simulink model "SyncGen_with_Grid_controll"  (R2013a)
settings: Solver=ode23  StartTime=2  StopTime=10  FixedStep=10^-3  MaxStep=1e-2  RelTol=1e-2
undefined symbols (not defined in the file): J, L_g, R_g, R_l
libraries: powerlib x18, powerlib_meascontrol x4, SyncGenLib x1
settings Model: Creator=Elad  LastModifiedBy=USER
settings DataIOCC: SignalLoggingSaveFormat=ModelDataLogs
settings DebuggingCC: MultiTaskDSMMsg=warning  MultiTaskCondExecSysMsg=none  StateNameClashWarn=none  StrictBusMsg=None
settings RTWCC: IncludeERTFirstTime=on

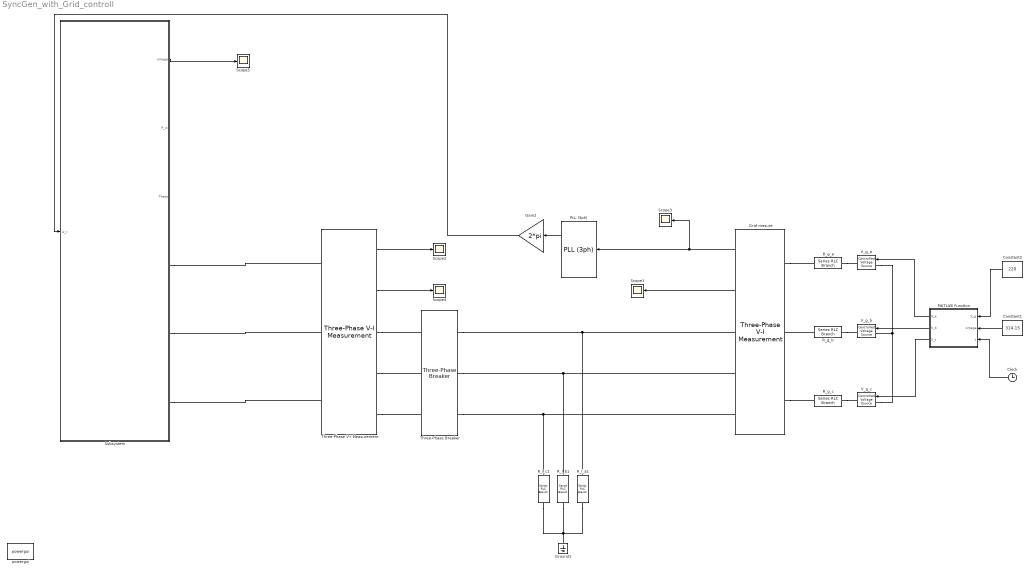
== system SyncGen_with_Grid_controll ==
  Clock : Clock
  Constant1 : Constant  Value=314.15
  Constant2 : Constant  Value=220
  Gain2 : Gain  Gain=2*pi
  Grid mesure : powerlib/Measurements/Three-Phase V-I Measurement  VoltageMeasurement=phase-to-ground  SetLabelV=off  LabelV=Vabc  Vpu=off  VpuLL=off  CurrentMeasurement=yes  SetLabelI=off  LabelI=Iabc  Ipu=off  Pbase=100e6  Vbase=500e3  OutputType=Complex  PhasorSimulation=off  PSBequivalent=0
  Ground1 : powerlib/Elements/Ground  LConnTagsString=a
  MATLAB Function : MATLAB Function  TreatAsAtomicUnit=on
  PLL (3ph) : powerlib_meascontrol/PLL/PLL (3ph)  Fmin=45  Par_Init=[0, 60]  ParK=[180, 3200, 1]  TcD=1e-4  MaxRateChangeFreq=12  FilterCutOffFreq=25  Ts=0  AGC=on
  R_g_a : powerlib/Elements/Series RLC Branch  LConnTagsString=__new0  RConnTagsString=__new0  BranchType=RL  Resistance=R_g  Inductance=L_g  SetiL0=off  InitialCurrent=0  Capacitance=1e-6  Setx0=off  InitialVoltage=0  Measurements=None
  R_g_b : powerlib/Elements/Series RLC Branch  LConnTagsString=__new0  RConnTagsString=__new0  BranchType=RL  Resistance=R_g  Inductance=L_g  SetiL0=off  InitialCurrent=0  Capacitance=1e-6  Setx0=off  InitialVoltage=0  Measurements=None
  R_g_c : powerlib/Elements/Series RLC Branch  LConnTagsString=__new0  RConnTagsString=__new0  BranchType=RL  Resistance=R_g  Inductance=L_g  SetiL0=off  InitialCurrent=0  Capacitance=1e-6  Setx0=off  InitialVoltage=0  Measurements=None
  R_l_a1 : powerlib/Elements/Series RLC Branch  LConnTagsString=__new0  RConnTagsString=__new0  BranchType=R  Resistance=R_l  Inductance=1e-3  SetiL0=off  InitialCurrent=0  Capacitance=1e-6  Setx0=off  InitialVoltage=0  Measurements=None
  R_l_b1 : powerlib/Elements/Series RLC Branch  LConnTagsString=__new0  RConnTagsString=__new0  BranchType=R  Resistance=R_l  Inductance=1e-3  SetiL0=off  InitialCurrent=0  Capacitance=1e-6  Setx0=off  InitialVoltage=0  Measurements=None
  R_l_c1 : powerlib/Elements/Series RLC Branch  LConnTagsString=__new0  RConnTagsString=__new0  BranchType=R  Resistance=R_l  Inductance=1e-3  SetiL0=off  InitialCurrent=0  Capacitance=1e-6  Setx0=off  InitialVoltage=0  Measurements=None
  Scope{1..5} (5 alike) : Scope
      Scope1 settings: TimeRange=5  YMin=-0.11  YMax=0.11
      Scope2 settings: TimeRange=8  YMin=-12.5  YMax=15
      Scope3 settings: TimeRange=5  YMin=-200  YMax=225  SaveName=ScopeData3
      Scope4 settings: TimeRange=5  YMin=-0.005  YMax=0.005  SaveName=ScopeData4
      Scope5 settings: TimeRange=5  YMin=293  YMax=316  SaveName=ScopeData2
  Subsystem : Subsystem
  Three-Phase V-I Measurement : powerlib/Measurements/Three-Phase V-I Measurement  VoltageMeasurement=phase-to-ground  SetLabelV=off  LabelV=Vabc  Vpu=off  VpuLL=off  CurrentMeasurement=yes  SetLabelI=off  LabelI=Iabc  Ipu=off  Pbase=100e6  Vbase=500e3  OutputType=Complex  PhasorSimulation=off  PSBequivalent=0
  Three-Phase Breaker : powerlib/Elements/Three-Phase Breaker  InitialState=open  SwitchA=on  SwitchB=on  SwitchC=on  SwitchTimes=[5]  External=off  BreakerResistance=0.001  SnubberResistance=1e6  SnubberCapacitance=inf  Measurements=None
  V_g_a : powerlib/Electrical Sources/Controlled Voltage Source  Initialize=off  Source_Type=AC  Amplitude=0  Phase=0  Frequency=0  Measurements=None
  V_g_b : powerlib/Electrical Sources/Controlled Voltage Source  Initialize=off  Source_Type=AC  Amplitude=0  Phase=0  Frequency=0  Measurements=None
  V_g_c : powerlib/Electrical Sources/Controlled Voltage Source  Initialize=off  Source_Type=AC  Amplitude=0  Phase=0  Frequency=0  Measurements=None
  powergui : powerlib/powergui  Priority=1  SimulationMode=Continuous  SolverType=Tustin  SampleTime=50e-6  frequency=60  SPID=off  DisableSnubberDevices=off  DisableRonSwitches=off  DisableVfSwitches=off  SwTol=0  Interpol=off  DisplayEquations=off  frequencyindice=0  Pbase=100e6  ErrMax=1e-4  Iterations=50  UnitsV=kV  UnitsW=MW  FunctionMessages=off  echomessages=off  HookPort=off  EnableUseOfTLC=off  x0status=blocks  RestoreLinks=warning  ResistiveCurrentMeasurement=off  Frange=[0:2:500]  Ylog=off  Xlog=on  ShowGrid=off  save=off  variable=ZData  ZoomFFT=off  StartTime=0.0  cycles=1  DisplayStyle=1  fundamental=60  FreqAxis=off  MaxFrequency=1000  frequencyindicesteady=1  RmsSteady=1  display=off  Ts=0  methode=off
  wires:
  Three-Phase V-I Measurement/1 -> Scope2/1
  Three-Phase V-I Measurement/2 -> Scope4/1
  Subsystem/1(omega) -> Scope5/1
  MATLAB Function/1(V_a) -> V_g_a/1
  MATLAB Function/2(V_b) -> V_g_b/1
  MATLAB Function/3(V_c) -> V_g_c/1
  Constant1/1 -> MATLAB Function/2(omega)
  Constant2/1 -> MATLAB Function/1(V_g)
  Clock/1 -> MATLAB Function/3(t)
  Grid mesure/2 -> Scope1/1
  Grid mesure/1 -> Scope3/1, PLL (3ph)/1
  PLL (3ph)/1 -> Gain2/1
  Gain2/1 -> Subsystem/1(w_r)
  connections:
  V_g_a/LConn1 -- V_g_b/LConn1 -- V_g_c/LConn1
  R_l_b1/RConn1 -- R_l_a1/RConn1 -- Ground1/LConn1 -- R_l_c1/RConn1
  Grid mesure/RConn2 -- Three-Phase Breaker/RConn2 -- R_l_b1/LConn1
  Grid mesure/RConn3 -- R_l_c1/LConn1 -- Three-Phase Breaker/RConn3
  R_g_b/LConn1 -- V_g_b/RConn1
  R_g_c/LConn1 -- V_g_c/RConn1
  Grid mesure/LConn1 -- R_g_a/RConn1
  R_g_a/LConn1 -- V_g_a/RConn1
  R_g_b/RConn1 -- Grid mesure/LConn2
  Grid mesure/LConn3 -- R_g_c/RConn1
  R_l_a1/LConn1 -- Grid mesure/RConn1 -- Three-Phase Breaker/RConn1
  Subsystem/RConn1 -- Three-Phase V-I Measurement/LConn1
  Subsystem/RConn2 -- Three-Phase V-I Measurement/LConn2
  Subsystem/RConn3 -- Three-Phase V-I Measurement/LConn3
  Three-Phase V-I Measurement/RConn1 -- Three-Phase Breaker/LConn1
  Three-Phase V-I Measurement/RConn2 -- Three-Phase Breaker/LConn2
  Three-Phase V-I Measurement/RConn3 -- Three-Phase Breaker/LConn3

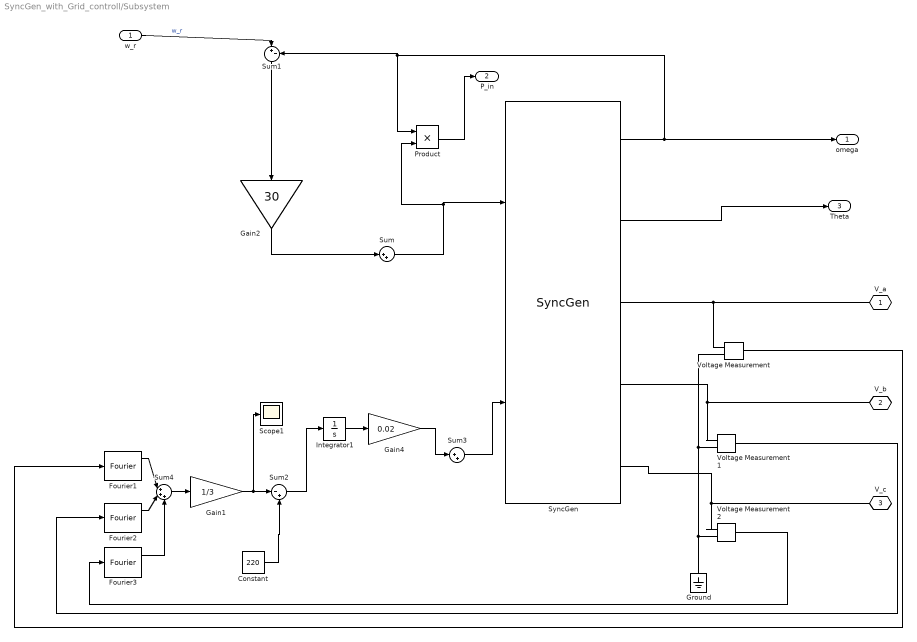
== system SyncGen_with_Grid_controll/Subsystem ==
  w_r : Inport
  Constant : Constant  Value=220
  Fourier1 : powerlib_meascontrol/Measurements/Fourier  Freq=60  n=1  InInit=[0, 0]  Ts=0
  Fourier2 : powerlib_meascontrol/Measurements/Fourier  Freq=60  n=1  InInit=[0, 0]  Ts=0
  Fourier3 : powerlib_meascontrol/Measurements/Fourier  Freq=60  n=1  InInit=[0, 0]  Ts=0
  Gain1 : Gain  Gain=1/3
  Gain2 : Gain  Gain=30
  Gain4 : Gain  Gain=0.02
  Ground : powerlib/Elements/Ground  LConnTagsString=a
  Integrator1 : Integrator
  Product : Product
  Scope1 : Scope
      settings: TimeRange=5  YMin=192.5  YMax=220  SaveName=ScopeData6
  Sum : Sum  Inputs=|++
  Sum1 : Sum  Inputs=|+-
  Sum2 : Sum  Inputs=|-+
  Sum3 : Sum  Inputs=|++
  Sum4 : Sum  Inputs=|+++
  "SyncGen " : SyncGenLib/SyncGen   R_f=R_f  R_s=R_s  D_p=D_p  J=J  M_f=M_f  L_f=L_f  L_s=L_s
  Voltage Measurement : powerlib/Measurements/Voltage Measurement  PhasorSimulation=off  OutputType=Complex  PSBequivalent=0
  Voltage Measurement1 : powerlib/Measurements/Voltage Measurement  PhasorSimulation=off  OutputType=Complex  PSBequivalent=0
  Voltage Measurement2 : powerlib/Measurements/Voltage Measurement  PhasorSimulation=off  OutputType=Complex  PSBequivalent=0
  V_a : PMIOPort  Tag=PMCPort  Port=1  Side=Right
  V_b : PMIOPort  Tag=PMCPort  Port=2  Side=Right
  V_c : PMIOPort  Tag=PMCPort  Port=3  Side=Right
  omega : Outport
  P_in : Outport  Port=2
  Theta : Outport  Port=3
  wires:
  "SyncGen "/1 -> Sum1/2, Product/1, omega/1
  Sum1/1 -> Gain2/1
  w_r/1 -> Sum1/1  "w_r"
  Voltage Measurement/1 -> Fourier1/1
  Voltage Measurement2/1 -> Fourier3/1
  Voltage Measurement1/1 -> Fourier2/1
  Sum4/1 -> Gain1/1
  Sum2/1 -> Integrator1/1
  Sum3/1 -> "SyncGen "/2
  Integrator1/1 -> Gain4/1
  Gain4/1 -> Sum3/1
  Product/1 -> P_in/1
  Sum/1 -> Product/2, "SyncGen "/1
  Gain2/1 -> Sum/1
  Constant/1 -> Sum2/2
  Fourier1/1 -> Sum4/1
  Fourier2/1 -> Sum4/2
  Fourier3/1 -> Sum4/3
  Gain1/1 -> Scope1/1, Sum2/1
  "SyncGen "/2 -> Theta/1
  connections:
  "SyncGen "/RConn1 -- V_a/RConn1 -- Voltage Measurement/LConn1
  Voltage Measurement2/LConn1 -- V_c/RConn1 -- "SyncGen "/RConn3
  Voltage Measurement1/LConn1 -- V_b/RConn1 -- "SyncGen "/RConn2
  Voltage Measurement2/LConn2 -- Ground/LConn1 -- Voltage Measurement1/LConn2 -- Voltage Measurement/LConn2

== matlab function SyncGen_with_Grid_controll/MATLAB Function ==
  data: V_g input; V_a output; omega input; t input; V_b output; V_c output
function [V_a,V_b,V_c] = fcn(V_g,omega,t)
V_a = V_g*sin(omega*t);
V_b = V_g*sin(omega*t - 2*pi/3);
V_c = V_g*sin(omega*t - 4*pi/3);
